simulink model "kalmanlinear_noiseadded"  (R2019b)
settings: Solver=VariableStepAuto  StartTime=0.0  StopTime=10.0  RelTol=1e-3
undefined symbols (not defined in the file or in its folder): Continuous, Time
libraries: ctrlSharedLib x9
settings Model: Creator=Bekircan Keceoglu  LastModifiedBy=Bekircan Keceoglu

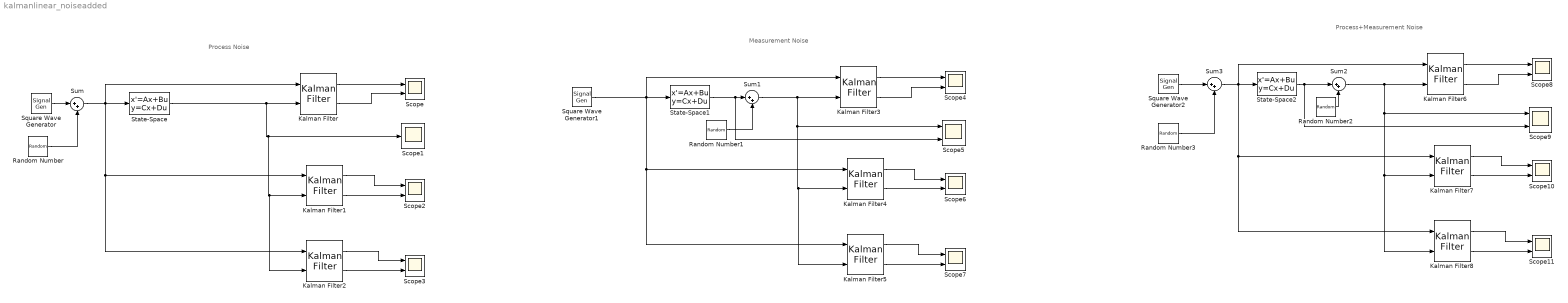
== system kalmanlinear_noiseadded ==
  note: Process Noise
  note: Measurement Noise
  note: Process+Measurement Noise
  Kalman Filter : ctrlSharedLib/Kalman Filter  TimeDomain=Continuous-Time  UseCurrentEstimator=on  ModelSource=Individual A, B, C, D matrices  ModelSourceVariable=ss(0.95,1,1,0,1)  A=[-1 -0.01; 1 0]  B=[1;0]  C=[0 1]  D=[0]  NumberOfStates=1  NumberOfInputs=1  NumberOfOutputs=1  InitialEstimateSource=Dialog  X0=0  P0=10  UseK=off  UseGH=off  NumberOfProcessNoiseInputs=1  G=1  TimeInvariantG=on  H=0  TimeInvariantH=on  Q=1  TimeInvariantQ=on  R=1  TimeInvariantR=on  N=0  TimeInvariantN=on  AddInputPort=on  AddEnablePort=off  OutputEstimatedY=on  OutputP=off  Ts=-1
      settings: SourceProductBaseCode=CT
  Kalman Filter1 : ctrlSharedLib/Kalman Filter  TimeDomain=Continuous-Time  UseCurrentEstimator=on  ModelSource=Individual A, B, C, D matrices  ModelSourceVariable=ss(0.95,1,1,0,1)  A=[-1 -0.01; 1 0]  B=[1;0]  C=[0 1]  D=[0]  NumberOfStates=1  NumberOfInputs=1  NumberOfOutputs=1  InitialEstimateSource=Dialog  X0=0  P0=10  UseK=off  UseGH=off  NumberOfProcessNoiseInputs=1  G=1  TimeInvariantG=on  H=0  TimeInvariantH=on  Q=10  TimeInvariantQ=on  R=0.1  TimeInvariantR=on  N=0  TimeInvariantN=on  AddInputPort=on  AddEnablePort=off  OutputEstimatedY=on  OutputP=off  Ts=-1
      settings: SourceProductBaseCode=CT
  Kalman Filter2 : ctrlSharedLib/Kalman Filter  TimeDomain=Continuous-Time  UseCurrentEstimator=on  ModelSource=Individual A, B, C, D matrices  ModelSourceVariable=ss(0.95,1,1,0,1)  A=[-1 -0.01; 1 0]  B=[1;0]  C=[0 1]  D=[0]  NumberOfStates=1  NumberOfInputs=1  NumberOfOutputs=1  InitialEstimateSource=Dialog  X0=0  P0=10  UseK=off  UseGH=off  NumberOfProcessNoiseInputs=1  G=1  TimeInvariantG=on  H=0  TimeInvariantH=on  Q=0.1  TimeInvariantQ=on  R=10  TimeInvariantR=on  N=0  TimeInvariantN=on  AddInputPort=on  AddEnablePort=off  OutputEstimatedY=on  OutputP=off  Ts=-1
      settings: SourceProductBaseCode=CT
  Kalman Filter3 : ctrlSharedLib/Kalman Filter  TimeDomain=Continuous-Time  UseCurrentEstimator=on  ModelSource=Individual A, B, C, D matrices  ModelSourceVariable=ss(0.95,1,1,0,1)  A=[-1 -0.01; 1 0]  B=[1;0]  C=[0 1]  D=[0]  NumberOfStates=1  NumberOfInputs=1  NumberOfOutputs=1  InitialEstimateSource=Dialog  X0=0  P0=10  UseK=off  UseGH=off  NumberOfProcessNoiseInputs=1  G=1  TimeInvariantG=on  H=0  TimeInvariantH=on  Q=1  TimeInvariantQ=on  R=1  TimeInvariantR=on  N=0  TimeInvariantN=on  AddInputPort=on  AddEnablePort=off  OutputEstimatedY=on  OutputP=off  Ts=-1
      settings: SourceProductBaseCode=CT
  Kalman Filter4 : ctrlSharedLib/Kalman Filter  TimeDomain=Continuous-Time  UseCurrentEstimator=on  ModelSource=Individual A, B, C, D matrices  ModelSourceVariable=ss(0.95,1,1,0,1)  A=[-1 -0.01; 1 0]  B=[1;0]  C=[0 1]  D=[0]  NumberOfStates=1  NumberOfInputs=1  NumberOfOutputs=1  InitialEstimateSource=Dialog  X0=0  P0=10  UseK=off  UseGH=off  NumberOfProcessNoiseInputs=1  G=1  TimeInvariantG=on  H=0  TimeInvariantH=on  Q=10  TimeInvariantQ=on  R=0.1  TimeInvariantR=on  N=0  TimeInvariantN=on  AddInputPort=on  AddEnablePort=off  OutputEstimatedY=on  OutputP=off  Ts=-1
      settings: SourceProductBaseCode=CT
  Kalman Filter5 : ctrlSharedLib/Kalman Filter  TimeDomain=Continuous-Time  UseCurrentEstimator=on  ModelSource=Individual A, B, C, D matrices  ModelSourceVariable=ss(0.95,1,1,0,1)  A=[-1 -0.01; 1 0]  B=[1;0]  C=[0 1]  D=[0]  NumberOfStates=1  NumberOfInputs=1  NumberOfOutputs=1  InitialEstimateSource=Dialog  X0=0  P0=10  UseK=off  UseGH=off  NumberOfProcessNoiseInputs=1  G=1  TimeInvariantG=on  H=0  TimeInvariantH=on  Q=0.1  TimeInvariantQ=on  R=10  TimeInvariantR=on  N=0  TimeInvariantN=on  AddInputPort=on  AddEnablePort=off  OutputEstimatedY=on  OutputP=off  Ts=-1
      settings: SourceProductBaseCode=CT
  Kalman Filter6 : ctrlSharedLib/Kalman Filter  TimeDomain=Continuous-Time  UseCurrentEstimator=on  ModelSource=Individual A, B, C, D matrices  ModelSourceVariable=ss(0.95,1,1,0,1)  A=[-1 -0.01; 1 0]  B=[1;0]  C=[0 1]  D=[0]  NumberOfStates=1  NumberOfInputs=1  NumberOfOutputs=1  InitialEstimateSource=Dialog  X0=0  P0=10  UseK=off  UseGH=off  NumberOfProcessNoiseInputs=1  G=1  TimeInvariantG=on  H=0  TimeInvariantH=on  Q=1  TimeInvariantQ=on  R=1  TimeInvariantR=on  N=0  TimeInvariantN=on  AddInputPort=on  AddEnablePort=off  OutputEstimatedY=on  OutputP=off  Ts=-1
      settings: SourceProductBaseCode=CT
  Kalman Filter7 : ctrlSharedLib/Kalman Filter  TimeDomain=Continuous-Time  UseCurrentEstimator=on  ModelSource=Individual A, B, C, D matrices  ModelSourceVariable=ss(0.95,1,1,0,1)  A=[-1 -0.01; 1 0]  B=[1;0]  C=[0 1]  D=[0]  NumberOfStates=1  NumberOfInputs=1  NumberOfOutputs=1  InitialEstimateSource=Dialog  X0=0  P0=10  UseK=off  UseGH=off  NumberOfProcessNoiseInputs=1  G=1  TimeInvariantG=on  H=0  TimeInvariantH=on  Q=10  TimeInvariantQ=on  R=0.1  TimeInvariantR=on  N=0  TimeInvariantN=on  AddInputPort=on  AddEnablePort=off  OutputEstimatedY=on  OutputP=off  Ts=-1
      settings: SourceProductBaseCode=CT
  Kalman Filter8 : ctrlSharedLib/Kalman Filter  TimeDomain=Continuous-Time  UseCurrentEstimator=on  ModelSource=Individual A, B, C, D matrices  ModelSourceVariable=ss(0.95,1,1,0,1)  A=[-1 -0.01; 1 0]  B=[1;0]  C=[0 1]  D=[0]  NumberOfStates=1  NumberOfInputs=1  NumberOfOutputs=1  InitialEstimateSource=Dialog  X0=0  P0=10  UseK=off  UseGH=off  NumberOfProcessNoiseInputs=1  G=1  TimeInvariantG=on  H=0  TimeInvariantH=on  Q=0.1  TimeInvariantQ=on  R=10  TimeInvariantR=on  N=0  TimeInvariantN=on  AddInputPort=on  AddEnablePort=off  OutputEstimatedY=on  OutputP=off  Ts=-1
      settings: SourceProductBaseCode=CT
  Random Number : RandomNumber  Mean=0.01  Variance=0.01  SampleTime=0.1
  Random Number1 : RandomNumber  Mean=0.01  Variance=0.01  SampleTime=0.1
  Random Number2 : RandomNumber  Mean=0.01  Variance=0.1  SampleTime=0.1
  Random Number3 : RandomNumber  Mean=0.01  Variance=0.01  SampleTime=0.1
  Scope{,2..11} (11 alike) : Scope  NumInputPorts=2
  Scope1 : Scope
  Square Wave Generator : SignalGenerator  WaveForm=square  Units=rad/sec
  Square Wave Generator1 : SignalGenerator  WaveForm=square  Units=rad/sec
  Square Wave Generator2 : SignalGenerator  WaveForm=square  Units=rad/sec
  State-Space : StateSpace  A=[-1 -0.01; 1 0]  B=[1; 0]  C=[0 1]  D=[0]  InitialCondition=[0 0]
  State-Space1 : StateSpace  A=[-1 -0.01; 1 0]  B=[1; 0]  C=[0 1]  D=[0]  InitialCondition=[0 0]
  State-Space2 : StateSpace  A=[-1 -0.01; 1 0]  B=[1; 0]  C=[0 1]  D=[0]  InitialCondition=[0 0]
  Sum{,1..3} (4 alike) : Sum  Inputs=|++
  wires:
  Kalman Filter1/1 -> Scope2/1
  Kalman Filter2/2 -> Scope3/2
  Kalman Filter2/1 -> Scope3/1
  Kalman Filter1/2 -> Scope2/2
  Kalman Filter/1 -> Scope/1
  Kalman Filter/2 -> Scope/2
  State-Space/1 -> Kalman Filter2/2, Kalman Filter1/2, Scope1/1, Kalman Filter/2
  Square Wave Generator/1 -> Sum/1
  Sum/1 -> Kalman Filter2/1, Kalman Filter1/1, Kalman Filter/1, State-Space/1
  Random Number/1 -> Sum/2
  Square Wave Generator1/1 -> Kalman Filter5/1, Kalman Filter4/1, Kalman Filter3/1, State-Space1/1
  Kalman Filter4/1 -> Scope6/1
  Kalman Filter3/1 -> Scope4/1
  Kalman Filter4/2 -> Scope6/2
  Kalman Filter5/1 -> Scope7/1
  Kalman Filter3/2 -> Scope4/2
  Kalman Filter5/2 -> Scope7/2
  State-Space1/1 -> Scope5/2, Sum1/1
  Sum1/1 -> Kalman Filter5/2, Kalman Filter4/2, Scope5/1, Kalman Filter3/2
  Random Number1/1 -> Sum1/2
  Kalman Filter6/2 -> Scope8/2
  Kalman Filter7/2 -> Scope10/2
  Kalman Filter6/1 -> Scope8/1
  Kalman Filter7/1 -> Scope10/1
  Random Number2/1 -> Sum2/2
  Sum2/1 -> Kalman Filter8/2, Kalman Filter7/2, Scope9/1, Kalman Filter6/2
  Kalman Filter8/1 -> Scope11/1
  Kalman Filter8/2 -> Scope11/2
  State-Space2/1 -> Scope9/2, Sum2/1
  Square Wave Generator2/1 -> Sum3/1
  Sum3/1 -> Kalman Filter8/1, Kalman Filter7/1, Kalman Filter6/1, State-Space2/1
  Random Number3/1 -> Sum3/2
